simulink model "ue_2_c"  (R2015b)
settings: Solver=VariableStepAuto  StartTime=0.0  StopTime=10  RelTol=1e-3
libraries: simulink x1
settings Model: Creator=dbarelop  LastModifiedBy=dbarelop

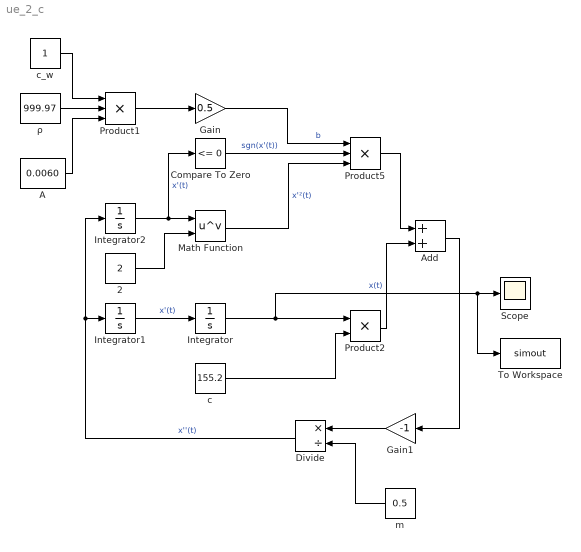
== system ue_2_c ==
  2 : Constant  Value=2
  A : Constant  Value=0.0060
  Add : Sum
  Compare To Zero : simulink/Logic and Bit Operations/Compare To Zero  relop=<=  OutDataTypeStr=uint8  ZeroCross=off
  Divide : Product  Inputs=*/
  Gain : Gain  Gain=0.5
  Gain1 : Gain  Gain=-1
  Integrator : Integrator  InitialCondition=1
  Integrator1 : Integrator
  Integrator2 : Integrator
  Math Function : Math  Operator=pow  SaturateOnIntegerOverflow=on
  Product1 : Product  Inputs=3
  Product2 : Product
  Product5 : Product  Inputs=3
  Scope : Scope
  To Workspace : ToWorkspace  VariableName=simout  SaveFormat=Timeseries  SampleTime=-1
  c : Constant  Value=155.2
  c_w : Constant
  m : Constant  Value=0.5
  ρ : Constant  Value=999.97
  wires:
  c_w/1 -> Product1/1
  Product1/1 -> Gain/1
  ρ/1 -> Product1/2
  Integrator1/1 -> Integrator/1  "x'(t)"
  2/1 -> Math Function/2
  Math Function/1 -> Product5/3  "x'²(t)"
  Integrator2/1 -> Compare To Zero/1, Math Function/1  "x'(t)"
  Compare To Zero/1 -> Product5/2  "sgn(x'(t))"
  Gain/1 -> Product5/1  "b"
  Add/1 -> Gain1/1
  Product5/1 -> Add/1
  Gain1/1 -> Divide/1
  A/1 -> Product1/3
  Integrator/1 -> To Workspace/1, Scope/1, Product2/1  "x(t)"
  c/1 -> Product2/2
  Product2/1 -> Add/2
  m/1 -> Divide/2
  Divide/1 -> Integrator2/1, Integrator1/1  "x''(t)"
